simulink model "s2dot3_56"  (R2023b)
settings: Solver=FixedStepAuto  StartTime=0.0  StopTime=1  FixedStep=0.1  RelTol=1e-3
settings Model: Creator=lxj  LastModifiedBy=lxj

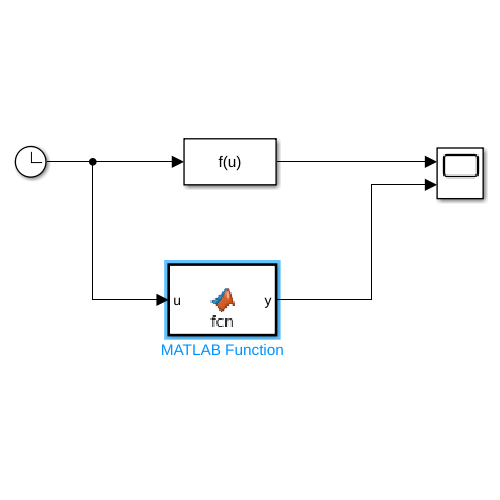
[thumbnail: Simulink's stored preview of the top-level diagram]
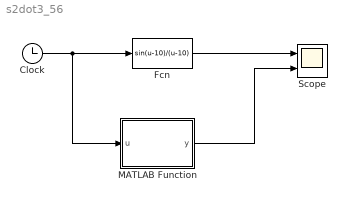
== system s2dot3_56 ==
  Clock : Clock
  Fcn : Fcn  Expr=sin(u-10)/(u-10)
  MATLAB Function : MATLAB Function  TreatAsAtomicUnit=on
  Scope : Scope  NumInputPorts=2
  wires:
  Clock/1 -> MATLAB Function/1(u), Fcn/1
  Fcn/1 -> Scope/1
  MATLAB Function/1(y) -> Scope/2

== matlab function s2dot3_56/MATLAB Function ==
  data: u input; y output
function y = fcn(u)
%#codegen
persistent sum_val;
if isempty(sum_val)
    sum_val = 0;
end
sum_val = sum_val + u;
y = sum_val;
